simulink model "open_closed_loop"  (R2022b)
settings: Solver=VariableStepAuto  StartTime=0.0  StopTime=20  RelTol=1e-3
settings Model: Creator=giuli  LastModifiedBy=giuli

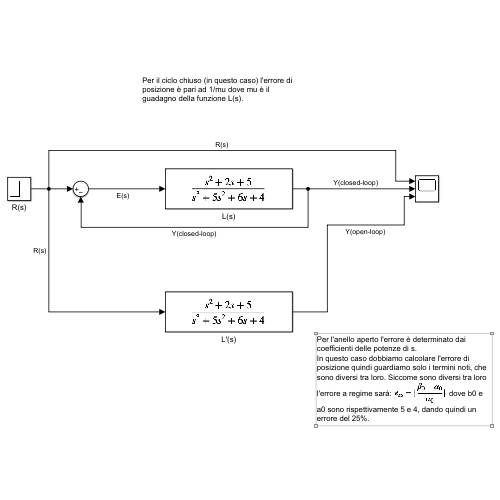
[thumbnail: Simulink's stored preview of the top-level diagram]
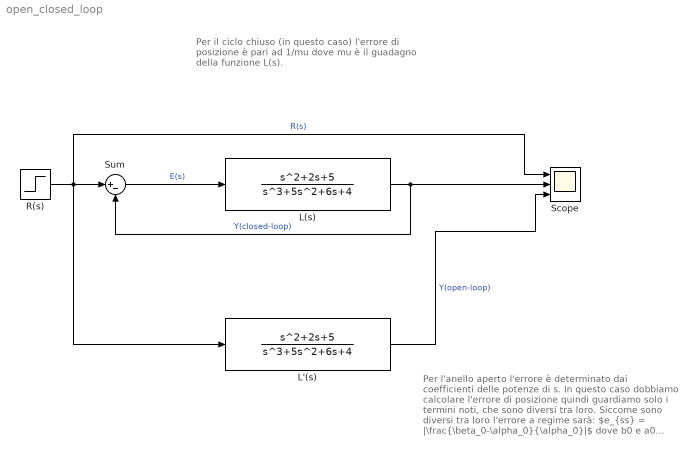
== system open_closed_loop ==
  note: Per l'anello aperto l'errore è determinato dai coefficienti delle potenze di s.
      | In questo caso dobbiamo calcolare l'errore di posizione quindi guardiamo solo i termini noti, che sono diversi tra loro. Siccome sono diversi tra loro l'errore a regime sarà: $e_{ss} = |\frac{\beta_0-\alpha_0}{\alpha_0}|$ dove b0 e a0 sono rispettivamente 5 e 4, dando quindi un errore del 25%.
  note: Per il ciclo chiuso (in questo caso) l'errore di posizione è pari ad 1/mu dove mu è il guadagno della funzione L(s).
  L'(s) : TransferFcn  Numerator=[1 2 5]  Denominator=[1 5 6 4]
  L(s) : TransferFcn  Numerator=[1 2 5]  Denominator=[1 5 6 4]
  R(s) : Step  SampleTime=0
  Scope : Scope  NumInputPorts=3
  Sum : Sum  Inputs=|+-
  wires:
  L(s)/1 -> Sum/2, Scope/2  "Y(closed-loop)"
  R(s)/1 -> Scope/1, L'(s)/1, Sum/1  "R(s)"
  L'(s)/1 -> Scope/3  "Y(open-loop)"
  Sum/1 -> L(s)/1  "E(s)"
